simulink model "BicycleHalfCarModel"  (R2020b)
settings: Solver=VariableStepAuto  StartTime=0.0  StopTime=10.0  RelTol=1e-3
settings Model: Creator=Authorized User  LastModifiedBy=Authorized User

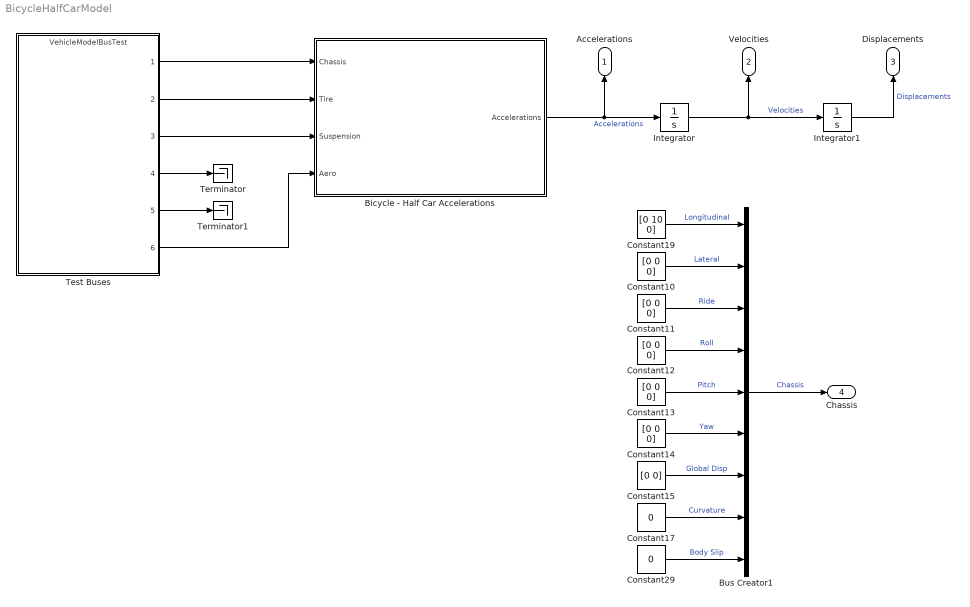
== system BicycleHalfCarModel ==
  Bicycle - Half Car Accelerations : MATLAB Function  TreatAsAtomicUnit=on
  Bus Creator1 : BusCreator  Inputs=9
  Constant{10..14} (5 alike) : Constant  Value=[0 0 0]
  Constant15 : Constant  Value=[0 0]
  Constant17 : Constant  Value=0
  Constant19 : Constant  Value=[0 10 0]
  Constant29 : Constant  Value=0
  Integrator : Integrator
  Integrator1 : Integrator
  Terminator : Terminator
  Terminator1 : Terminator
  Test Buses : ModelReference  ModelNameDialog=VehicleModelBusTest.slx  SimulationMode=Normal  ModelReferenceVersion=1.30
  Accelerations : Outport
  Velocities : Outport  Port=2
  Displacements : Outport  Port=3
  Chassis : Outport  Port=4  OutDataTypeStr=Bus: Chassis
  wires:
  Bicycle - Half Car Accelerations/1(Accelerations) -> Accelerations/1, Integrator/1  "Accelerations"
  Integrator/1 -> Velocities/1, Integrator1/1  "Velocities"
  Integrator1/1 -> Displacements/1  "Displacements"
  Test Buses/6 -> Bicycle - Half Car Accelerations/4(Aero)
  Test Buses/3 -> Bicycle - Half Car Accelerations/3(Suspension)
  Test Buses/2 -> Bicycle - Half Car Accelerations/2(Tire)
  Test Buses/4 -> Terminator/1
  Test Buses/5 -> Terminator1/1
  Test Buses/1 -> Bicycle - Half Car Accelerations/1(Chassis)
  Constant12/1 -> Bus Creator1/4  "Roll"
  Bus Creator1/1 -> Chassis/1  "Chassis"
  Constant29/1 -> Bus Creator1/9  "Body Slip"
  Constant14/1 -> Bus Creator1/6  "Yaw"
  Constant15/1 -> Bus Creator1/7  "Global Disp"
  Constant11/1 -> Bus Creator1/3  "Ride"
  Constant13/1 -> Bus Creator1/5  "Pitch"
  Constant19/1 -> Bus Creator1/1  "Longitudinal"
  Constant17/1 -> Bus Creator1/8  "Curvature"
  Constant10/1 -> Bus Creator1/2  "Lateral"

== matlab function BicycleHalfCarModel/Bicycle - Half Car Accelerations ==
  data: Chassis input; Accelerations output; Tire input; Suspension input; Aero input
function Accelerations = Acceleration_Evaluation( Chassis, Tire, Suspension, Aero )

y = u;
